simulink model "BlockV3"  (R2017a)
settings: Solver=VariableStepAuto  StartTime=0.0  StopTime=Tsim  FixedStep=0.001  RelTol=1e-3
values from neighbouring files (symbols this model uses):
  b = 0.1    [Model_old.m]
  g = 40    [Model_old.m]    (also in ModeloBase_OLD.m)
  J = 0.01    [Model_old.m]
  Kd = 0    [Model_old.m]
  Ke = 0.08    [Model_old.m]
  Ki = 10.0    (= 10)    [Model_old.m]
  Kp = 5.0    (= 5)    [Model_old.m]
  ksi = 0.6    [Model_old.m]    (also in ModeloBase_OLD.m = 0.3)
  L = 0.5    [Model_old.m]
  R = 1    [Model_old.m]
  Ts = 0.1    [Model_old.m]    (also in ModeloBase_OLD.m; PIController.m)
  Ts_sensor = 1/50    (= 0.02)    [Model_old.m]
undefined symbols (not defined in the file or in its folder): DiscIntNeverNeededParam, F_M, Ts_compute
libraries: simulink x16, cstblocks x6, simulink_extras x2
settings Model: Creator=davi2  LastModifiedBy=davi2

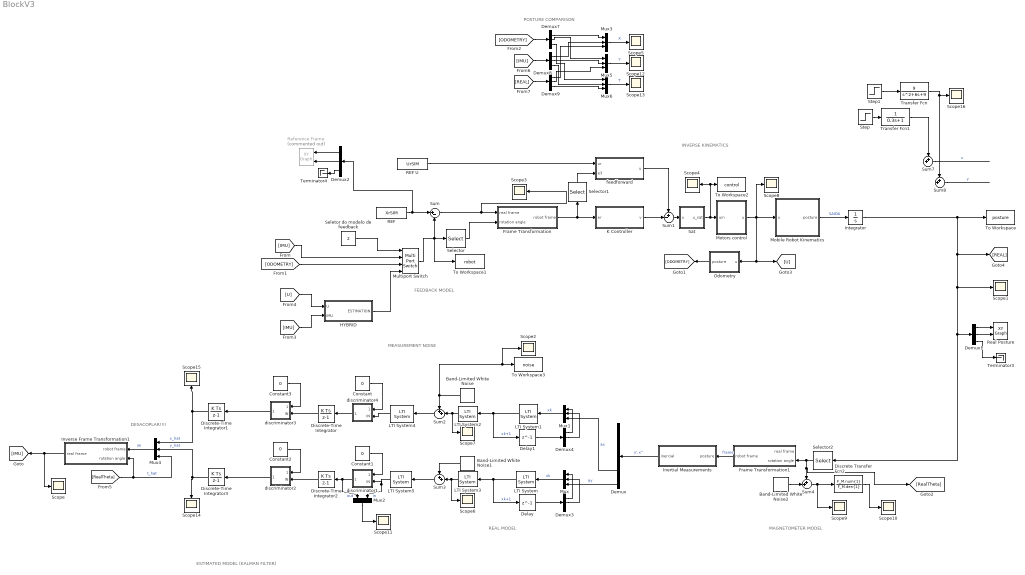
== system BlockV3 ==
  note: DESACOPLAR!!!!
  note: POSTURE COMPARISON
  note: MEASUREMENT NOISE
  note: REAL MODEL
  note: INVERSE KINEMATICS
  note: MAGNETOMETER MODEL
  note: FEEDBACK MODEL
  note: ESTIMATED MODEL (KALMAN FILTER)
  Band-Limited White Noise : simulink/Sources/Band-Limited White Noise  Cov=0.00001  Ts=Ts_sensor  seed=[23341]
  Band-Limited White Noise1 : simulink/Sources/Band-Limited White Noise  Cov=0.00001  Ts=Ts_sensor  seed=[23341]
  Band-Limited White Noise2 : simulink/Sources/Band-Limited White Noise  Cov=0.00001  Ts=1/200  seed=[23341]
  Constant{,1..3} (4 alike) : Constant  Value=0
  Delay : Delay  DelayLength=1
  Delay1 : Delay  DelayLength=1
  Demux : Demux  Outputs=5
  Demux{1..4,7..9} (7 alike) : Demux  Outputs=3
  Discrete Transfer Fcn2 : DiscreteTransferFcn  Numerator=F_M.num{1}  Denominator=F_M.den{1}
  Discrete-Time Integrator{,1..3} (4 alike) : DiscreteIntegrator  InitialConditionSetting=State (most efficient)  SampleTime=Ts_sensor  ICPrevOutput=DiscIntNeverNeededParam  ICPrevScaledInput=DiscIntNeverNeededParam
  Frame Transformation : Subsystem
  Frame Transformation1 : Subsystem
  HYBRID : Subsystem
  Inertial Measurements : Subsystem
  Integrator : Integrator
  Inverse Frame Transformation1 : Subsystem
  K Controller : Subsystem
  LTI System : cstblocks/LTI System  sys=A  IC=[]
  LTI System1 : cstblocks/LTI System  sys=A  IC=[]
  LTI System2 : cstblocks/LTI System  sys=C  IC=[]
  LTI System3 : cstblocks/LTI System  sys=C  IC=[]
  LTI System4 : cstblocks/LTI System  sys=F_M  IC=[]
  LTI System5 : cstblocks/LTI System  sys=F_M  IC=[]
  Mobile Robot Kinematics : Subsystem
  Motors control : Subsystem
  Multiport Switch : MultiPortSwitch
  Mux{,1,3..6} (6 alike) : Mux  Inputs=3
  Mux2 : Mux  Inputs=2
  Odometry : Subsystem
  REF : FromWorkspace  VariableName=XrSIM  SampleTime=Ts  OutputAfterFinalValue=Holding final value
  REF U : FromWorkspace  VariableName=UrSIM  SampleTime=Ts  OutputAfterFinalValue=Holding final value
  Real Posture : simulink/Sinks/XY Graph  xmin=0  xmax=3  ymin=-0.8  ymax=1.5  st=Ts
  Reference Frame : simulink/Sinks/XY Graph  Commented=on  xmin=0  xmax=2  ymin=0  ymax=1.5  st=Ts
  Sat : Subsystem
  Scope{,1..16} (17 alike) : Scope
  Selector : Selector  InputPortWidth=3  IndexOptions=Index vector (dialog)  Indices=3  OutputSizes=1
  Selector1 : Selector  InputPortWidth=3  IndexOptions=Index vector (dialog)  Indices=3  OutputSizes=1
  Selector2 : Selector  InputPortWidth=3  IndexOptions=Index vector (dialog)  Indices=3  OutputSizes=1
  Seletor do modelo de feedback : Constant  Value=2
  Step : Step  Time=20  After=0  SampleTime=0
  Step1 : Step  Time=5  After=-0.4  SampleTime=0
  Sum : Sum  Inputs=|+-
  Sum1 : Sum  Inputs=+-|
  Sum{2..4,7..8} (5 alike) : Sum  Inputs=++|
  Terminator3 : Terminator
  Terminator4 : Terminator
  To Workspace : ToWorkspace  VariableName=posture  SaveFormat=Timeseries  SampleTime=-1
  To Workspace1 : ToWorkspace  VariableName=robot  SaveFormat=Timeseries  SampleTime=-1
  To Workspace2 : ToWorkspace  VariableName=control  SaveFormat=Timeseries  SampleTime=-1
  To Workspace3 : ToWorkspace  VariableName=noise  SaveFormat=Timeseries  SampleTime=-1
  Transfer Fcn : TransferFcn  Numerator=9  Denominator=[1 6 9]
  Transfer Fcn1 : TransferFcn  Denominator=[0.3 1]
  discriminator1 : Subsystem
  discriminator2 : Subsystem
  discriminator3 : Subsystem
  discriminator4 : Subsystem
  feedforward : Subsystem
  wires:
  Sum/1 -> Scope3/1, Frame Transformation/1(real frame)
  Selector/1 -> Frame Transformation/2(rotation angle)
  Frame Transformation/1(robot frame) -> K Controller/1(er), Selector1/1
  REF U/1 -> feedforward/1(ur)
  Selector1/1 -> feedforward/2(e3)
  feedforward/1(u) -> Sum1/1
  K Controller/1(v) -> Sum1/2
  Motors control/1(u) -> Odometry/1(u), [U], Mobile Robot Kinematics/1(u), Scope8/1
  Selector2/1 -> Frame Transformation1/2(rotation angle), [RealTheta], Sum4/1
  Frame Transformation1/1(robot frame) -> Inertial Measurements/1(posture)  "frame"
  Demux1/1 -> Real Posture/1
  Demux1/2 -> Real Posture/2
  REF/1 -> Demux2/1, Sum/1
  [IMU] -> Multiport Switch/2
  [ODOMETRY] -> Multiport Switch/3
  Odometry/1(posture) -> [ODOMETRY]
  Sum1/1 -> Sat/1(u)
  Sat/1(u_sat) -> Scope4/1, To Workspace2/1, Motors control/1(uin)
  Multiport Switch/1 -> Sum/2, Selector/1, To Workspace1/1
  Demux1/3 -> Terminator3/1
  Seletor do modelo de feedback/1 -> Multiport Switch/1
  HYBRID/1(ESTIMATION) -> Multiport Switch/4
  [IMU] -> HYBRID/2(IMU)
  [U] -> HYBRID/1(U)
  Band-Limited White Noise2/1 -> Sum4/2
  Sum4/1 -> Discrete Transfer Fcn2/1, Scope9/1
  Discrete Transfer Fcn2/1 -> Scope10/1
  Demux2/1 -> Reference Frame/1
  Demux2/2 -> Reference Frame/2
  Demux2/3 -> Terminator4/1
  Inertial Measurements/1(inercial) -> Demux/1  "x',x''"
  LTI System/1 -> LTI System3/1, Delay/1  "xk+1"
  Delay/1 -> Demux3/1
  Demux3/1 -> Mux/1
  Demux3/2 -> Mux/2
  Demux/5 -> Mux/3  "ay"
  Mux/1 -> LTI System/1  "xk"
  Demux4/2 -> Mux1/2
  Delay1/1 -> Demux4/1
  Demux/4 -> Mux1/3  "ax"
  Demux4/1 -> Mux1/1
  LTI System1/1 -> Delay1/1, LTI System2/1  "xk+1"
  Mux1/1 -> LTI System1/1  "xk"
  Inverse Frame Transformation1/1(real frame) -> [IMU], Scope/1
  [RealTheta] -> Mux4/3, Inverse Frame Transformation1/2(rotation angle)  "t_hat"
  LTI System2/1 -> Scope7/1, Sum2/2
  Band-Limited White Noise1/1 -> Sum3/1
  LTI System3/1 -> Scope6/1, Sum3/2
  Mux4/1 -> Inverse Frame Transformation1/1(robot frame)  "im"
  Band-Limited White Noise/1 -> Scope2/1, To Workspace3/1, Sum2/1
  [REAL] -> Demux9/1
  [ODOMETRY] -> Demux7/1
  [IMU] -> Demux8/1
  Demux7/1 -> Mux3/1
  Demux8/1 -> Mux3/2
  Demux7/2 -> Mux5/1
  Demux8/2 -> Mux5/2
  Demux9/2 -> Mux5/3
  Demux7/3 -> Mux6/1
  Demux8/3 -> Mux6/2
  Demux9/3 -> Mux6/3
  Mux3/1 -> Scope5/1  "X"
  Mux5/1 -> Scope12/1  "Y"
  Mux6/1 -> Scope13/1  "T"
  Discrete-Time Integrator1/1 -> Mux4/1, Scope15/1  "x_hat"
  Discrete-Time Integrator3/1 -> Scope14/1, Mux4/2  "y_hat"
  Sum2/1 -> LTI System4/1
  Sum3/1 -> LTI System5/1
  LTI System5/1 -> discriminator1/2(IN), Mux2/2  "in"
  discriminator1/1(OUT) -> Mux2/1, Discrete-Time Integrator2/1  "out"
  Mux2/1 -> Scope11/1
  Demux9/1 -> Mux3/3
  LTI System4/1 -> discriminator4/2(IN)
  discriminator4/1(OUT) -> Discrete-Time Integrator/1
  Constant/1 -> discriminator4/1(value)
  Constant1/1 -> discriminator1/1(value)
  Discrete-Time Integrator/1 -> discriminator3/2(IN)
  Discrete-Time Integrator2/1 -> discriminator2/2(IN)
  discriminator2/1(OUT) -> Discrete-Time Integrator3/1
  discriminator3/1(OUT) -> Discrete-Time Integrator1/1
  Constant3/1 -> discriminator3/1(value)
  Constant2/1 -> discriminator2/1(value)
  Sum8/1 -> ?  "y"
  Step1/1 -> Transfer Fcn/1
  Transfer Fcn1/1 -> Sum7/1
  Sum7/1 -> ?  "x"
  Transfer Fcn/1 -> Sum8/1, Scope16/1
  ? -> Sum7/2
  Step/1 -> Transfer Fcn1/1
  ? -> Sum8/2
  Mobile Robot Kinematics/1(posture) -> Integrator/1  "SAIDA"
  Integrator/1 -> Selector2/1, Demux1/1, Scope1/1, [REAL], To Workspace/1

== system BlockV3/Frame Transformation ==
  real frame : Inport
  rotation angle : Inport  Port=2
  Mux : Mux  Inputs=2
  S-Function : S-Function  FunctionName=Real2Robot  Parameters=Ts  SFunctionDeploymentMode=off  EnableBusSupport=off
  robot frame : Outport
  wires:
  real frame/1 -> Mux/1
  rotation angle/1 -> Mux/2
  Mux/1 -> S-Function/1
  S-Function/1 -> robot frame/1

== system BlockV3/Frame Transformation1 ==
  real frame : Inport
  rotation angle : Inport  Port=2
  Mux : Mux  Inputs=2
  S-Function : S-Function  FunctionName=Real2Robot  Parameters=Ts_compute  SFunctionDeploymentMode=off  EnableBusSupport=off
  robot frame : Outport
  wires:
  real frame/1 -> Mux/1
  rotation angle/1 -> Mux/2
  Mux/1 -> S-Function/1
  S-Function/1 -> robot frame/1

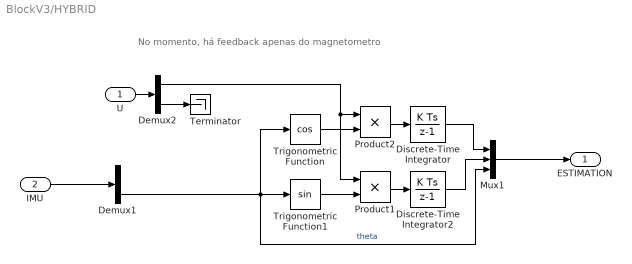
== system BlockV3/HYBRID ==
  note: No momento, há feedback apenas do magnetometro
  U : Inport
  IMU : Inport  Port=2
  Demux1 : Demux  Outputs=3
  Demux2 : Demux  Outputs=2
  Discrete-Time Integrator : DiscreteIntegrator  InitialConditionSetting=State (most efficient)  SampleTime=Ts  ICPrevOutput=DiscIntNeverNeededParam  ICPrevScaledInput=DiscIntNeverNeededParam
  Discrete-Time Integrator2 : DiscreteIntegrator  InitialConditionSetting=State (most efficient)  SampleTime=Ts  ICPrevOutput=DiscIntNeverNeededParam  ICPrevScaledInput=DiscIntNeverNeededParam
  Mux1 : Mux  Inputs=3
  Product1 : Product
  Product2 : Product
  Terminator : Terminator
  Trigonometric Function : Trigonometry  Operator=cos
  Trigonometric Function1 : Trigonometry
  ESTIMATION : Outport
  wires:
  IMU/1 -> Demux1/1
  Trigonometric Function1/1 -> Product1/2
  Demux2/1 -> Product1/1, Product2/1
  Trigonometric Function/1 -> Product2/2
  Product2/1 -> Discrete-Time Integrator/1
  Discrete-Time Integrator/1 -> Mux1/1
  Discrete-Time Integrator2/1 -> Mux1/2
  Demux1/3 -> Mux1/3, Trigonometric Function/1, Trigonometric Function1/1  "theta"
  Product1/1 -> Discrete-Time Integrator2/1
  Mux1/1 -> ESTIMATION/1
  U/1 -> Demux2/1
  Demux2/2 -> Terminator/1

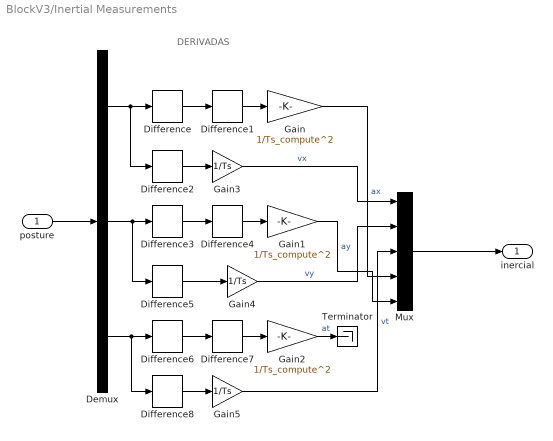
== system BlockV3/Inertial Measurements ==
  note: DERIVADAS
  posture : Inport
  Demux : Demux  Outputs=3
  Difference{,1..8} (9 alike) : simulink/Discrete/Difference  ICPrevInput=0.0  OutMin=[]  OutMax=[]  OutDataType=fixdt(1, 16)  OutScaling=2^-10  DoSatur=off
  Gain : Gain  Gain=1/Ts_compute^2
  Gain1 : Gain  Gain=1/Ts_compute^2
  Gain2 : Gain  Gain=1/Ts_compute^2
  Gain3 : Gain  Gain=1/Ts
  Gain4 : Gain  Gain=1/Ts
  Gain5 : Gain  Gain=1/Ts
  Mux : Mux  Inputs=5
  Terminator : Terminator
  inercial : Outport
  wires:
  posture/1 -> Demux/1
  Difference/1 -> Difference1/1
  Difference3/1 -> Difference4/1
  Difference6/1 -> Difference7/1
  Demux/3 -> Difference8/1, Difference6/1
  Demux/2 -> Difference5/1, Difference3/1
  Demux/1 -> Difference2/1, Difference/1
  Difference1/1 -> Gain/1
  Difference4/1 -> Gain1/1
  Difference7/1 -> Gain2/1
  Difference2/1 -> Gain3/1
  Difference8/1 -> Gain5/1
  Difference5/1 -> Gain4/1
  Mux/1 -> inercial/1
  Gain3/1 -> Mux/1  "vx"
  Gain4/1 -> Mux/2  "vy"
  Gain5/1 -> Mux/3  "vt"
  Gain/1 -> Mux/4  "ax"
  Gain1/1 -> Mux/5  "ay"
  Gain2/1 -> Terminator/1  "at"

== system BlockV3/Inverse Frame Transformation1 ==
  robot frame : Inport
  rotation angle : Inport  Port=2
  Mux : Mux  Inputs=2
  S-Function : S-Function  FunctionName=Robot2Real  Parameters=Ts  SFunctionDeploymentMode=off  EnableBusSupport=off
  real frame : Outport
  wires:
  S-Function/1 -> real frame/1
  Mux/1 -> S-Function/1
  rotation angle/1 -> Mux/2
  robot frame/1 -> Mux/1

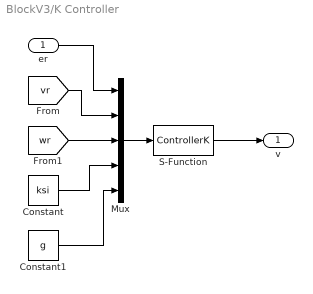
== system BlockV3/K Controller ==
  er : Inport
  Constant : Constant  Value=ksi
  Constant1 : Constant  Value=g
  Mux : Mux  Inputs=5
  S-Function : S-Function  FunctionName=ControllerK  Parameters=Ts  SFunctionDeploymentMode=off  EnableBusSupport=off
  v : Outport
  wires:
  er/1 -> Mux/1
  [vr] -> Mux/2
  [wr] -> Mux/3
  Constant/1 -> Mux/4
  Constant1/1 -> Mux/5
  Mux/1 -> S-Function/1
  S-Function/1 -> v/1

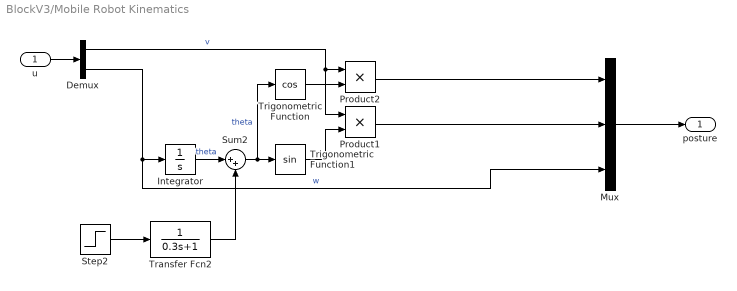
== system BlockV3/Mobile Robot Kinematics ==
  u : Inport
  Demux : Demux  Outputs=2
  Integrator : Integrator
  Mux : Mux  Inputs=3
  Product1 : Product
  Product2 : Product
  Step2 : Step  Time=5  After=0  SampleTime=0
  Sum2 : Sum  Inputs=|++
  Transfer Fcn2 : TransferFcn  Denominator=[0.3 1]
  Trigonometric Function : Trigonometry  Operator=cos
  Trigonometric Function1 : Trigonometry
  posture : Outport
  wires:
  u/1 -> Demux/1
  Demux/2 -> Mux/3, Integrator/1  "w"
  Trigonometric Function/1 -> Product2/2
  Demux/1 -> Product1/1, Product2/1  "v"
  Product2/1 -> Mux/1
  Trigonometric Function1/1 -> Product1/2
  Product1/1 -> Mux/2
  Mux/1 -> posture/1
  Step2/1 -> Transfer Fcn2/1
  Integrator/1 -> Sum2/1  "theta"
  Sum2/1 -> Trigonometric Function/1, Trigonometric Function1/1  "theta"
  Transfer Fcn2/1 -> Sum2/2

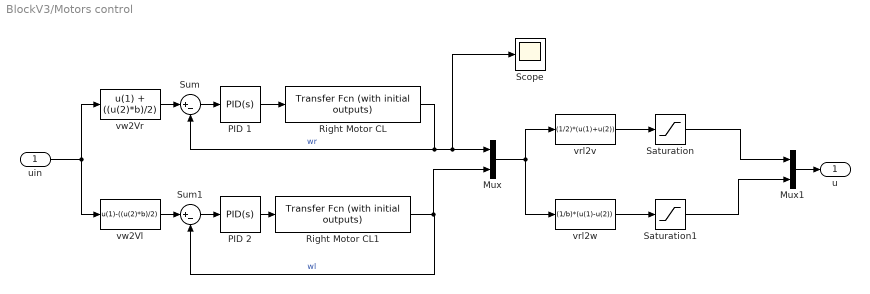
== system BlockV3/Motors control ==
  uin : Inport
  Mux : Mux  Inputs=2
  Mux1 : Mux  Inputs=2
  PID 1 : simulink/Continuous/PID Controller  Controller=PID  TimeDomain=Continuous-time  SampleTime=-1  IntegratorMethod=Forward Euler  FilterMethod=Forward Euler  Form=Parallel  UseFilter=on  ControllerParametersSource=internal  P=Kp  I=Ki  D=Kd  N=100  InitialConditionSource=internal  InitialConditionForIntegrator=0  InitialConditionForFilter=0  ExternalReset=none  LimitOutput=off  UpperSaturationLimit=inf  LowerSaturationLimit=-inf  LinearizeAsGain=on  AntiWindupMode=none  Kb=1  TrackingMode=off  Kt=1  PParamMin=[]  PParamMax=[]  IParamMin=[]  IParamMax=[]  DParamMin=[]  DParamMax=[]  NParamMin=[]  NParamMax=[]  KbParamMin=[]  KbParamMax=[]  KtParamMin=[]  KtParamMax=[]  POutMin=[]  POutMax=[]  IOutMin=[]  IOutMax=[]  DOutMin=[]  DOutMax=[]  NOutMin=[]  NOutMax=[]  KbOutMin=[]  KbOutMax=[]  KtOutMin=[]  KtOutMax=[]  IntegratorOutMin=[]  IntegratorOutMax=[]  FilterOutMin=[]  FilterOutMax=[]  SumOutMin=[]  SumOutMax=[]  SumI1OutMin=[]  SumI1OutMax=[]  SumI2OutMin=[]  SumI2OutMax=[]  SumI3OutMin=[]  SumI3OutMax=[]  SumDOutMin=[]  SumDOutMax=[]  SaturationOutMin=[]  SaturationOutMax=[]  IntegratorContinuousStateAttributes=''  IntegratorStateMustResolveToSignalObject=off  IntegratorRTWStateStorageClass=Auto  FilterContinuousStateAttributes=''  FilterStateMustResolveToSignalObject=off  FilterRTWStateStorageClass=Auto  DifferentiatorICPrevScaledInput=0  DifferentiatorOutMin=[]  DifferentiatorOutMax=[]  InitialConditionSetting=State (most efficient)
  PID 2 : simulink/Continuous/PID Controller  Controller=PID  TimeDomain=Continuous-time  SampleTime=-1  IntegratorMethod=Forward Euler  FilterMethod=Forward Euler  Form=Parallel  UseFilter=on  ControllerParametersSource=internal  P=Kp  I=Ki  D=Kd  N=100  InitialConditionSource=internal  InitialConditionForIntegrator=0  InitialConditionForFilter=0  ExternalReset=none  LimitOutput=off  UpperSaturationLimit=inf  LowerSaturationLimit=-inf  LinearizeAsGain=on  AntiWindupMode=none  Kb=1  TrackingMode=off  Kt=1  PParamMin=[]  PParamMax=[]  IParamMin=[]  IParamMax=[]  DParamMin=[]  DParamMax=[]  NParamMin=[]  NParamMax=[]  KbParamMin=[]  KbParamMax=[]  KtParamMin=[]  KtParamMax=[]  POutMin=[]  POutMax=[]  IOutMin=[]  IOutMax=[]  DOutMin=[]  DOutMax=[]  NOutMin=[]  NOutMax=[]  KbOutMin=[]  KbOutMax=[]  KtOutMin=[]  KtOutMax=[]  IntegratorOutMin=[]  IntegratorOutMax=[]  FilterOutMin=[]  FilterOutMax=[]  SumOutMin=[]  SumOutMax=[]  SumI1OutMin=[]  SumI1OutMax=[]  SumI2OutMin=[]  SumI2OutMax=[]  SumI3OutMin=[]  SumI3OutMax=[]  SumDOutMin=[]  SumDOutMax=[]  SaturationOutMin=[]  SaturationOutMax=[]  IntegratorContinuousStateAttributes=''  IntegratorStateMustResolveToSignalObject=off  IntegratorRTWStateStorageClass=Auto  FilterContinuousStateAttributes=''  FilterStateMustResolveToSignalObject=off  FilterRTWStateStorageClass=Auto  DifferentiatorICPrevScaledInput=0  DifferentiatorOutMin=[]  DifferentiatorOutMax=[]  InitialConditionSetting=State (most efficient)
  Right Motor CL : simulink_extras/Additional Linear/Transfer Fcn (with initial outputs)  N=[Ke]  D="[J*L  (J*R+b*L) (b*R+Ke^2)]"  Y0=0  U0=0
  Right Motor CL1 : simulink_extras/Additional Linear/Transfer Fcn (with initial outputs)  N=[Ke]  D="[J*L  (J*R+b*L) (b*R+Ke^2)]"  Y0=0  U0=0
  Saturation : Saturate  UpperLimit=1  LowerLimit=-1
  Saturation1 : Saturate  UpperLimit=1  LowerLimit=-1
  Scope : Scope
  Sum : Sum  Inputs=|+-
  Sum1 : Sum  Inputs=|+-
  vrl2v : Fcn  Expr=(1/2)*(u(1)+u(2))
  vrl2w : Fcn  Expr=(1/b)*(u(1)-u(2))
  vw2Vl : Fcn  Expr=u(1)-((u(2)*b)/2)
  vw2Vr : Fcn  Expr=u(1) + ((u(2)*b)/2)
  u : Outport
  wires:
  vw2Vr/1 -> Sum/1
  Right Motor CL1/1 -> Mux/2, Sum1/2  "wl"
  vw2Vl/1 -> Sum1/1
  Sum1/1 -> PID 2/1
  PID 2/1 -> Right Motor CL1/1
  Sum/1 -> PID 1/1
  PID 1/1 -> Right Motor CL/1
  Right Motor CL/1 -> Mux/1, Scope/1, Sum/2  "wr"
  uin/1 -> vw2Vl/1, vw2Vr/1
  Mux/1 -> vrl2v/1, vrl2w/1
  Mux1/1 -> u/1
  vrl2w/1 -> Saturation1/1
  vrl2v/1 -> Saturation/1
  Saturation/1 -> Mux1/1
  Saturation1/1 -> Mux1/2

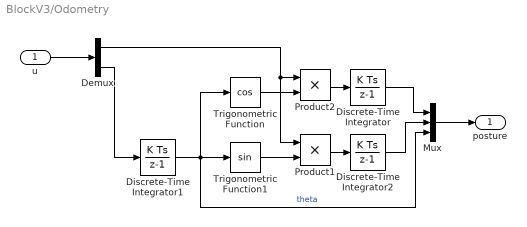
== system BlockV3/Odometry ==
  u : Inport
  Demux : Demux  Outputs=2
  Discrete-Time Integrator : DiscreteIntegrator  InitialConditionSetting=State (most efficient)  SampleTime=Ts  ICPrevOutput=DiscIntNeverNeededParam  ICPrevScaledInput=DiscIntNeverNeededParam
  Discrete-Time Integrator1 : DiscreteIntegrator  InitialConditionSetting=State (most efficient)  SampleTime=Ts  ICPrevOutput=DiscIntNeverNeededParam  ICPrevScaledInput=DiscIntNeverNeededParam
  Discrete-Time Integrator2 : DiscreteIntegrator  InitialConditionSetting=State (most efficient)  SampleTime=Ts  ICPrevOutput=DiscIntNeverNeededParam  ICPrevScaledInput=DiscIntNeverNeededParam
  Mux : Mux  Inputs=3
  Product1 : Product
  Product2 : Product
  Trigonometric Function : Trigonometry  Operator=cos
  Trigonometric Function1 : Trigonometry
  posture : Outport
  wires:
  u/1 -> Demux/1
  Demux/2 -> Discrete-Time Integrator1/1
  Discrete-Time Integrator1/1 -> Mux/3, Trigonometric Function/1, Trigonometric Function1/1  "theta"
  Trigonometric Function/1 -> Product2/2
  Demux/1 -> Product1/1, Product2/1
  Product2/1 -> Discrete-Time Integrator/1
  Trigonometric Function1/1 -> Product1/2
  Product1/1 -> Discrete-Time Integrator2/1
  Discrete-Time Integrator/1 -> Mux/1
  Discrete-Time Integrator2/1 -> Mux/2
  Mux/1 -> posture/1

== system BlockV3/Sat ==
  u : Inport
  Demux : Demux  Outputs=2
  Mux : Mux  Inputs=2
  Saturation : Saturate  LowerLimit=0
  Saturation1 : Saturate
  u_sat : Outport
  wires:
  Demux/2 -> Saturation1/1  "W"
  Demux/1 -> Saturation/1  "V"
  u/1 -> Demux/1
  Saturation/1 -> Mux/1
  Saturation1/1 -> Mux/2
  Mux/1 -> u_sat/1

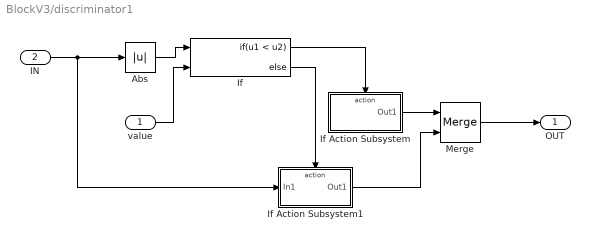
== system BlockV3/discriminator1 ==
  value : Inport
  IN : Inport  Port=2
  Abs : Abs
  If : If  NumInputs=2  IfExpression=u1 < u2
  If Action Subsystem : Subsystem  TreatAsAtomicUnit=on
  If Action Subsystem1 : Subsystem  TreatAsAtomicUnit=on
  Merge : Merge
  OUT : Outport
  wires:
  IN/1 -> If Action Subsystem1/1(In1), Abs/1
  Abs/1 -> If/1
  If/1 -> If Action Subsystem/Action
  If/2 -> If Action Subsystem1/Action
  If Action Subsystem/1(Out1) -> Merge/1
  If Action Subsystem1/1(Out1) -> Merge/2
  Merge/1 -> OUT/1
  value/1 -> If/2

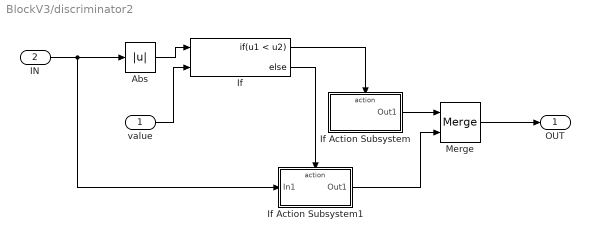
== system BlockV3/discriminator2 ==
  value : Inport
  IN : Inport  Port=2
  Abs : Abs
  If : If  NumInputs=2  IfExpression=u1 < u2
  If Action Subsystem : Subsystem  TreatAsAtomicUnit=on
  If Action Subsystem1 : Subsystem  TreatAsAtomicUnit=on
  Merge : Merge
  OUT : Outport
  wires:
  IN/1 -> If Action Subsystem1/1(In1), Abs/1
  Abs/1 -> If/1
  If/1 -> If Action Subsystem/Action
  If/2 -> If Action Subsystem1/Action
  If Action Subsystem/1(Out1) -> Merge/1
  If Action Subsystem1/1(Out1) -> Merge/2
  Merge/1 -> OUT/1
  value/1 -> If/2

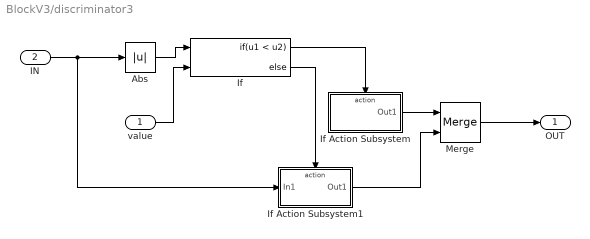
== system BlockV3/discriminator3 ==
  value : Inport
  IN : Inport  Port=2
  Abs : Abs
  If : If  NumInputs=2  IfExpression=u1 < u2
  If Action Subsystem : Subsystem  TreatAsAtomicUnit=on
  If Action Subsystem1 : Subsystem  TreatAsAtomicUnit=on
  Merge : Merge
  OUT : Outport
  wires:
  IN/1 -> If Action Subsystem1/1(In1), Abs/1
  Abs/1 -> If/1
  If/1 -> If Action Subsystem/Action
  If/2 -> If Action Subsystem1/Action
  If Action Subsystem/1(Out1) -> Merge/1
  If Action Subsystem1/1(Out1) -> Merge/2
  Merge/1 -> OUT/1
  value/1 -> If/2

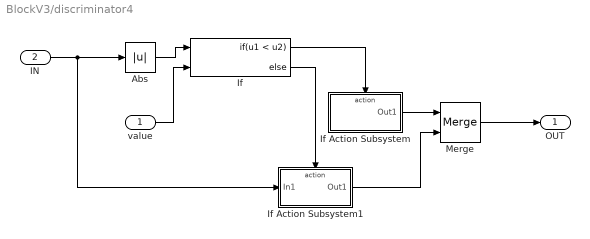
== system BlockV3/discriminator4 ==
  value : Inport
  IN : Inport  Port=2
  Abs : Abs
  If : If  NumInputs=2  IfExpression=u1 < u2
  If Action Subsystem : Subsystem  TreatAsAtomicUnit=on
  If Action Subsystem1 : Subsystem  TreatAsAtomicUnit=on
  Merge : Merge
  OUT : Outport
  wires:
  IN/1 -> If Action Subsystem1/1(In1), Abs/1
  Abs/1 -> If/1
  If/1 -> If Action Subsystem/Action
  If/2 -> If Action Subsystem1/Action
  If Action Subsystem/1(Out1) -> Merge/1
  If Action Subsystem1/1(Out1) -> Merge/2
  Merge/1 -> OUT/1
  value/1 -> If/2

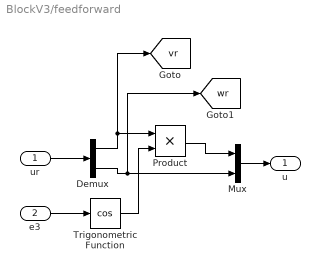
== system BlockV3/feedforward ==
  ur : Inport
  e3 : Inport  Port=2
  Demux : Demux  Outputs=2
  Mux : Mux  Inputs=2
  Product : Product
  Trigonometric Function : Trigonometry  Operator=cos
  u : Outport
  tag scope: vr=global, wr=global
  wires:
  e3/1 -> Trigonometric Function/1
  ur/1 -> Demux/1
  Demux/1 -> [vr], Product/1
  Trigonometric Function/1 -> Product/2
  Product/1 -> Mux/1
  Demux/2 -> [wr], Mux/2
  Mux/1 -> u/1

== system BlockV3/discriminator1/If Action Subsystem ==
  Action Port : ActionPort  ActionType=then
  Constant : Constant  Value=0
  Out1 : Outport
  wires:
  Constant/1 -> Out1/1

== system BlockV3/discriminator1/If Action Subsystem1 ==
  In1 : Inport
  Action Port : ActionPort  ActionType=else
  Out1 : Outport
  wires:
  In1/1 -> Out1/1

== system BlockV3/discriminator2/If Action Subsystem ==
  Action Port : ActionPort  ActionType=then
  Constant : Constant  Value=0
  Out1 : Outport
  wires:
  Constant/1 -> Out1/1

== system BlockV3/discriminator2/If Action Subsystem1 ==
  In1 : Inport
  Action Port : ActionPort  ActionType=else
  Out1 : Outport
  wires:
  In1/1 -> Out1/1

== system BlockV3/discriminator3/If Action Subsystem ==
  Action Port : ActionPort  ActionType=then
  Constant : Constant  Value=0
  Out1 : Outport
  wires:
  Constant/1 -> Out1/1

== system BlockV3/discriminator3/If Action Subsystem1 ==
  In1 : Inport
  Action Port : ActionPort  ActionType=else
  Out1 : Outport
  wires:
  In1/1 -> Out1/1

== system BlockV3/discriminator4/If Action Subsystem ==
  Action Port : ActionPort  ActionType=then
  Constant : Constant  Value=0
  Out1 : Outport
  wires:
  Constant/1 -> Out1/1

== system BlockV3/discriminator4/If Action Subsystem1 ==
  In1 : Inport
  Action Port : ActionPort  ActionType=else
  Out1 : Outport
  wires:
  In1/1 -> Out1/1
